simulink model "trajectory_IMU"  (R2021a)
settings: Solver=VariableStepAuto  StartTime=0.0  StopTime=tf  RelTol=1e-3
values from neighbouring files (symbols this model uses):
  misalignment_ax = R_yaw_ref*R_pitch_ax*R_roll_ax    [imu_params.m]
  misalignment_ref = R_yaw_ref*R_pitch_ref*R_roll_ref    [imu_params.m]
libraries: dspstat3 x3
settings Model: Creator=Laura  LastModifiedBy=Laura

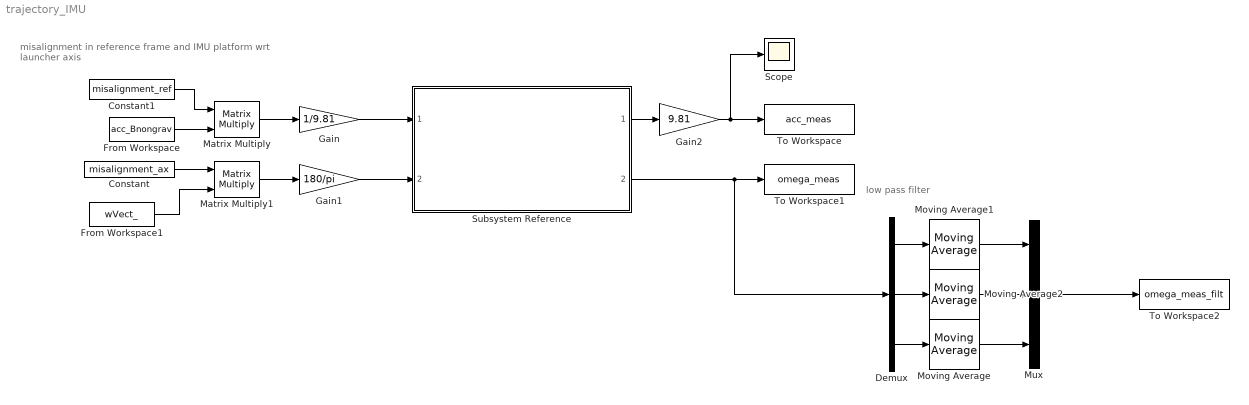
== system trajectory_IMU ==
  note: low pass filter
  note: misalignment in reference frame and
      | IMU platform wrt launcher axis
  Constant : Constant  Value=misalignment_ax
  Constant1 : Constant  Value=misalignment_ref
  Demux : Demux  Outputs=3
  From Workspace : FromWorkspace  VariableName=acc_Bnongrav
  From Workspace1 : FromWorkspace  VariableName=wVect_
  Gain : Gain  Gain=1/9.81
  Gain1 : Gain  Gain=180/pi
  Gain2 : Gain  Gain=9.81
  Matrix Multiply : Product  Multiplication=Matrix(*)
  Matrix Multiply1 : Product  Multiplication=Matrix(*)
  Moving Average : dspstat3/Moving Average  Method=Sliding window  ForgettingFactorPort=off  SpecifyWindowLength=on  WindowLength=14000  ForgettingFactor=0.9  SimulateUsing=Code generation
  Moving Average1 : dspstat3/Moving Average  Method=Sliding window  ForgettingFactorPort=on  SpecifyWindowLength=on  WindowLength=14000  ForgettingFactor=0.9  SimulateUsing=Code generation
  Moving Average2 : dspstat3/Moving Average  Method=Sliding window  ForgettingFactorPort=off  SpecifyWindowLength=on  WindowLength=14000  ForgettingFactor=0.9  SimulateUsing=Code generation
  Mux : Mux  Inputs=3
  Scope : Scope
  Subsystem Reference : Subsystem  ReferencedSubsystem=IMU
  To Workspace : ToWorkspace  VariableName=acc_meas  SaveFormat=Timeseries  SampleTime=-1
  To Workspace1 : ToWorkspace  VariableName=omega_meas  SaveFormat=Timeseries  SampleTime=-1
  To Workspace2 : ToWorkspace  VariableName=omega_meas_filt  SaveFormat=Timeseries  SampleTime=-1
  wires:
  Subsystem Reference/1 -> Gain2/1
  Gain/1 -> Subsystem Reference/1
  Subsystem Reference/2 -> To Workspace1/1, Demux/1
  Demux/3 -> Moving Average/1
  Gain1/1 -> Subsystem Reference/2
  Demux/1 -> Moving Average1/1
  Demux/2 -> Moving Average2/1
  Moving Average1/1 -> Mux/1
  Moving Average2/1 -> Mux/2
  Moving Average/1 -> Mux/3
  Mux/1 -> To Workspace2/1
  Gain2/1 -> Scope/1, To Workspace/1
  From Workspace1/1 -> Matrix Multiply1/2
  From Workspace/1 -> Matrix Multiply/2
  Matrix Multiply/1 -> Gain/1
  Matrix Multiply1/1 -> Gain1/1
  Constant1/1 -> Matrix Multiply/1
  Constant/1 -> Matrix Multiply1/1
